simulink model "simu1_3"  (R2023a)
settings: Solver=VariableStepAuto  StartTime=0.0  StopTime=10.0  RelTol=1e-3
values from neighbouring files (symbols this model uses):
  b = 1.5    [mat1_3.m]
  g = 9.81    [mat1_3.m]
  k = 20    [mat1_3.m]
  m = 3    [mat1_3.m]
settings Model: Creator=lukas  LastModifiedBy=lukas

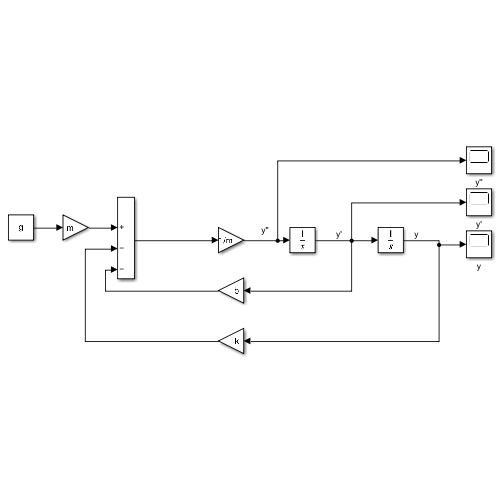
[thumbnail: Simulink's stored preview of the top-level diagram]
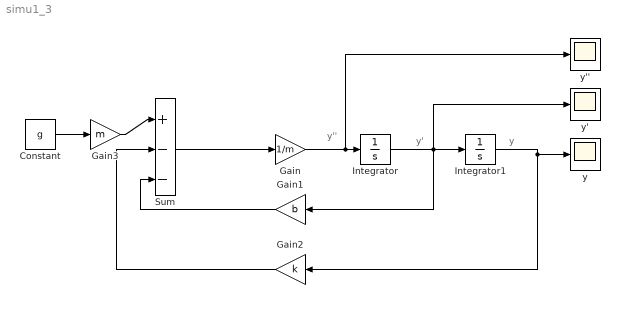
== system simu1_3 ==
  note: y
  note: y'
  note: y''
  Constant : Constant  Value=g
  Gain : Gain  Gain=1/m
  Gain1 : Gain  Gain=b
  Gain2 : Gain  Gain=k
  Gain3 : Gain  Gain=m
  Integrator : Integrator
  Integrator1 : Integrator
  Sum : Sum  Inputs=|+--
  y : Scope
  y' : Scope
  y'' : Scope
  wires:
  Integrator/1 -> y'/1, Gain1/1, Integrator1/1
  Integrator1/1 -> y/1, Gain2/1
  Gain/1 -> y''/1, Integrator/1
  Sum/1 -> Gain/1
  Constant/1 -> Gain3/1
  Gain3/1 -> Sum/1
  Gain2/1 -> Sum/2
  Gain1/1 -> Sum/3
